simulink model "simu_gyak3"  (R2023a)
settings: Solver=VariableStepAuto  StartTime=0.0  StopTime=10  RelTol=1e-3
settings Model: Creator=simon  LastModifiedBy=simon

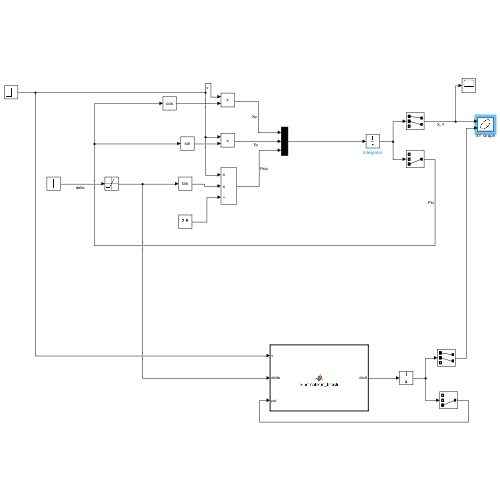
[thumbnail: Simulink's stored preview of the top-level diagram]
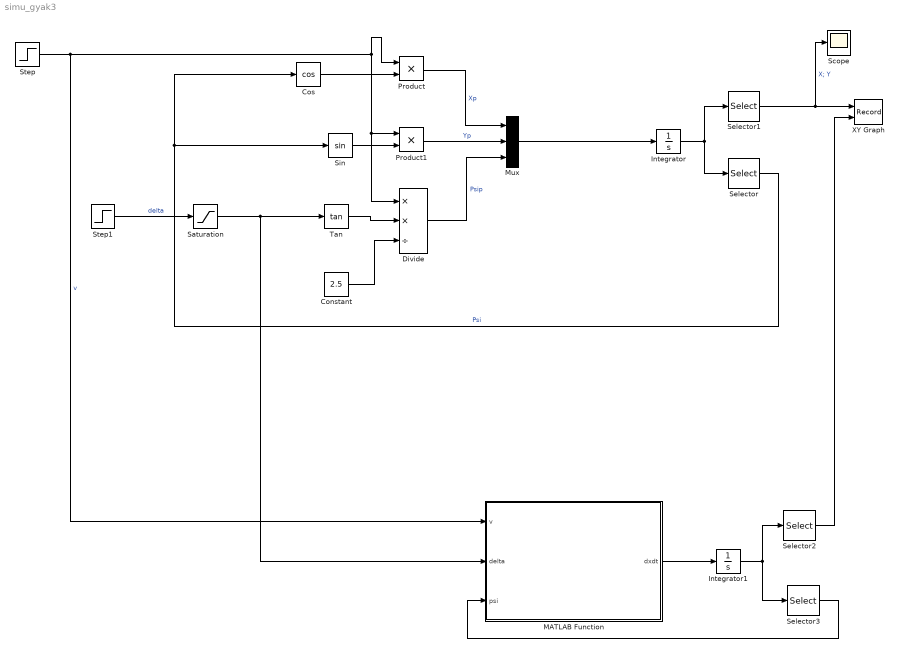
== system simu_gyak3 ==
  Constant : Constant  Value=2.5
  Cos : Trigonometry  Operator=cos
  Divide : Product  Inputs=**/
  Integrator : Integrator  InitialCondition=[0; 0; pi/3]
  Integrator1 : Integrator  InitialCondition=[-1; -1; pi/6]
  MATLAB Function : MATLAB Function  TreatAsAtomicUnit=on
  Mux : Mux  Inputs=3
  Product : Product
  Product1 : Product
  Saturation : Saturate
  Scope : Scope
  Selector : Selector  InputPortWidth=3  IndexOptions=Index vector (dialog)  Indices=3  OutputSizes=1
  Selector1 : Selector  InputPortWidth=3  IndexOptions=Index vector (dialog)  Indices=[1 2]  OutputSizes=1
  Selector2 : Selector  InputPortWidth=3  IndexOptions=Index vector (dialog)  Indices=[1 2]  OutputSizes=1
  Selector3 : Selector  InputPortWidth=3  IndexOptions=Index vector (dialog)  Indices=3  OutputSizes=1
  Sin : Trigonometry
  Step : Step  After=3  SampleTime=0
  Step1 : Step  Time=5  After=0.5  SampleTime=0
  Tan : Trigonometry  Operator=tan
  XY Graph : Record  FileSettingsInternal="{\"entries\":[{\"content\":{\"excelSettings\":{\"content\":{},\"type\":\"Streamout.ExcelSettings\"}},\"type\":\"Streamout.FileSettingStorage\",\"uuid\":\"\"}],\"packageUris\":[\"http:\\/\\/schema.mathworks.com\\/mf0\\/streamout_blocks\\/R2020a\"],\"version\":\"1.0\"}"  Layout=[1 1]  SignalsInternal="{\"entries\":[{\"content\":{\"signals\":[{\"content\":{\"blockPath\":[],\"dimensions\":[2],\"domain\":\"\",\"hasChildren\":true,\"lineColor\":\"#77ac30\",\"port\":1,\"sid\":[\"\"],\"signalID\":576,\"signalName\":\"X; Y\"},\"type\":\"RecordBlkView.Signal\",\"uuid\":\"\"},{\"content\":{\"blockPath\":[],\"channel\":[1],\"dimensions\":[2],\"domain\":\"\",\"lineColor\":\"#7e2f8e\",\"parentID\":576,\"plots\":[1],\"port\":1,\"sid\":[\"\"],\"signalID\":577,\"signalName\":\"X; Y\"},\"type\":\"RecordBlkView.Signal\",\"uuid\":\"\"},{\"content\":{\"blockPath\":[],\"dimensions\":[2,1],\"domain\":\"\",\"hasChildren\":true,\"lineColor\":\"#a2142f\",\"port\":2,\"sid\":[\"\"],\"signalID\":581,\"signalName\":\"Selector2\"},\"type\":\"RecordBlkView.Signal\",\"uuid\":\"\"},{\"content\":{\"blockPath\":[],\"channel\":[1,1],\"dimensions\":[2,1],\"domain\":\"\",\"lineColor\":\"#ff13a6\",\"parentID\":581,\"plots\":[1],\"port\":2,\"sid\":[\"\"],\"signalID\":582,\"signalName\":\"Selector2\"},\"type\":\"RecordBlkView.Signal\",\"uuid\":\"\"},{\"content\":{\"blockPath\":[],\"channel\":[2],\"dimensions\":[2],\"domain\":\"\",\"lineColor\":\"#a2142f\",\"parentID\":576,\"plots\":[1],\"port\":1,\"sid\":[\"\"],\"signalID\":586,\"signalName\":\"X; Y\"},\"type\":\"RecordBlkView.Signal\",\"uuid\":\"\"},{\"content\":{\"blockPath\":[],\"channel\":[2,1],\"dimensions\":[2,1],\"domain\":\"\",\"lineColor\":\"#22b573\",\"parentID\":581,\"plots\":[1],\"port\":2,\"sid\":[\"\"],\"signalID\":587,\"signalName\":\"Selector2\"},\"type\":\"RecordBlkView.Signal\",\"uuid\":\"\"}]},\"type\":\"RecordBlkView.InputSignals\",\"uuid\":\"\"}],\"packageUris\":[\"http:\\/\\/schema.mathworks.com\\/mf0\\/streamout_blocks\\/R2020a\"],\"version\":\"1.0\"}"  VisualizationBindings="{\"xyplotplugin\":{\"info\":[{\"series\":[{\"bindingParametersList\":[{\"parameter\":\"X-Axis\",\"signalID\":582,\"signalName\":\"Selector2(1,1)\"},{\"parameter\":\"Y-Axis\",\"signalID\":587,\"signalName\":\"Selector2(2,1)\"}],\"seriesID\":45900},{\"bindingParametersList\":[{\"parameter\":\"X-Axis\",\"signalID\":577,\"signalName\":\"X; Y(1)\"},{\"parameter\":\"Y-Axis\",\"signalID\":586,\"signalName\":\"X; Y(2)\"}],\"seriesID\":537}],\"subplotID\":1}]}}"  CompatibilityTag=XY
  wires:
  Tan/1 -> Divide/2
  Constant/1 -> Divide/3
  Product/1 -> Mux/1  "Xp"
  Product1/1 -> Mux/2  "Yp"
  Divide/1 -> Mux/3  "Psip"
  Mux/1 -> Integrator/1
  Step/1 -> MATLAB Function/1(v), Product/1, Divide/1, Product1/1  "v"
  Step1/1 -> Saturation/1  "delta"
  Integrator/1 -> Selector1/1, Selector/1
  Selector/1 -> Cos/1, Sin/1  "Psi"
  Selector1/1 -> XY Graph/1, Scope/1  "X; Y"
  Sin/1 -> Product1/2
  Cos/1 -> Product/2
  Saturation/1 -> MATLAB Function/2(delta), Tan/1
  MATLAB Function/1(dxdt) -> Integrator1/1
  Integrator1/1 -> Selector2/1, Selector3/1
  Selector3/1 -> MATLAB Function/3(psi)
  Selector2/1 -> XY Graph/2

== matlab function simu_gyak3/MATLAB Function ==
  data: v input; dxdt output; delta input; psi input
function dxdt = kinematikus_bicikli(v, delta, psi)

l = 2.5;
dxdt = [v*cos(psi); v*sin(psi); v*tan(delta)/l]
